simulink model "SystemModel"  (R2026a)
settings: Solver=FixedStepDiscrete  StopTime=inf  FixedStep=ts_system  EnableMultiTasking=on
StartFcn:
  | Simulink.sdi.setRecordData(false);
undefined symbols (not defined in the file): Battery, BCE12, BCE_Set_init, BMS_Controller_State, Cell10_P, Cell11_P, Cell12_P, Cell1_N, Cell1_P, Cell2_P, Cell3_P, Cell4_P, Cell5_P, Cell6_P, Cell7_P, Cell8_P, Cell9_P, Cell_Temperatures, Cell_Voltages, Charging_State, currentFactor, CV_Gain, Device_01, DiscIntNeverNeededParam, I_cc, MaxCellVoltThrsld, noCurrent, Ns_Module, NumModules, OverCellVoltageLimit, sg_bce, SOCInit, SRE, ts_controller, ts_system, UnderCellVoltageLimit, voltThreshold
libraries: slrealtimeethercatlib x99, fl_lib x65, nesl_utility x43, simulink x23, slrealtimeutilitieslib x13, sl_discontinuities x13, dspstat3 x12, canmsglib x11, speedgoatlib_IO611 x9, batt_lib x3, sharedTrackingLibrary x2, BatteryModuleLibrary_12Cells_lib x1
(part 6 of 6)

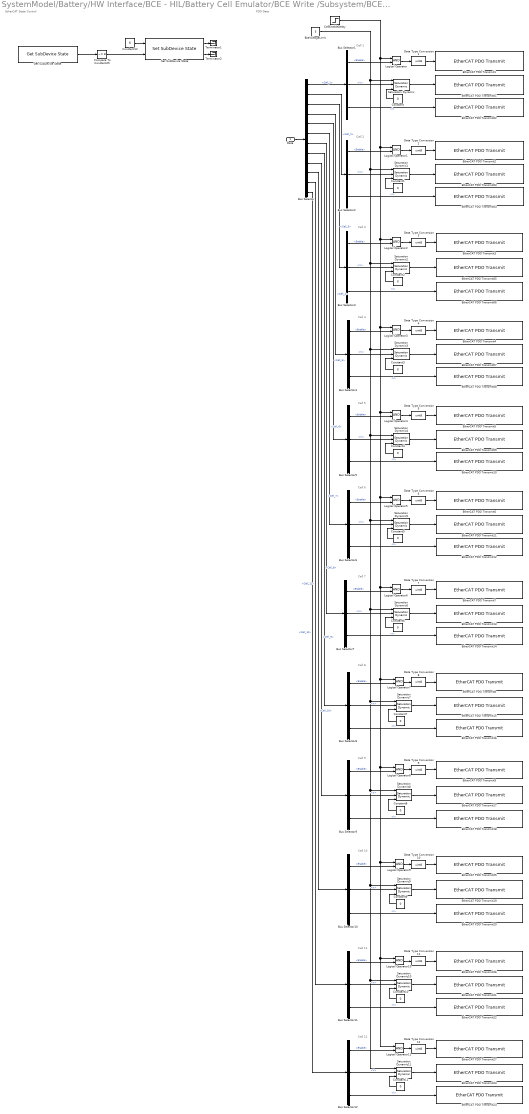
== system SystemModel/Battery/HW Interface/BCE - HIL/Battery Cell Emulator/BCE Write /Subsystem/BCE Write  ==
  note: EtherCAT State Control
  note: Cell 4
  note: Cell 8
  note: Cell 9
  note: Cell 1
  note: Cell 7
  note: PDO Data
  note: Cell 5
  note: Cell 3
  note: Cell 10
  note: Cell 6
  note: Cell 11
  note: Cell 12
  note: Cell 2
  Data : Inport  OutDataTypeStr=Bus: BCE_Set
  BceVoltageLimit : Constant  Value=5  SampleTime=0.001
  Bus Selector : BusSelector  OutputSignals=Cell_1,Cell_2,Cell_3,Cell_4,Cell_5,Cell_6,Cell_7,Cell_8,Cell_9,Cell_10,Cell_11,Cell_12
  Bus Selector{1..12} (12 alike) : BusSelector  OutputSignals=Enable,V,I
  CellEnableDelay : Step  Time=2  SampleTime=0.001
  Compare To Constant25 : simulink/Logic and Bit Operations/Compare To Constant  relop=~=  const=8  OutDataTypeStr=boolean
  Constant{,1..11} (12 alike) : Constant  Value=0
  Constant12 : Constant  Value=8  OutDataTypeStr=int32
  Data Type Conversion{1..12} (12 alike) : DataTypeConversion  OutDataTypeStr=uint8  SaturateOnIntegerOverflow=off  RndMeth=Floor
  EtherCAT PDO Transmit01 : slrealtimeethercatlib/EtherCAT PDO Transmit  Priority=3  sig_name=Device_01 (BCE12-0505).Rx_Cell_01.setVoltage  sig_offset=8  sig_type=single  type_size=32  sig_dim=1  device_id=0  sample_time=0.001000
  EtherCAT PDO Transmit02 : slrealtimeethercatlib/EtherCAT PDO Transmit  Priority=3  sig_name=Device_01 (BCE12-0505).Rx_Cell_01.setCurrent  sig_offset=40  sig_type=single  type_size=32  sig_dim=1  device_id=0  sample_time=0.001000
  EtherCAT PDO Transmit03 : slrealtimeethercatlib/EtherCAT PDO Transmit  Priority=3  sig_name=Device_01 (BCE12-0505).Rx_Cell_02.setVoltage  sig_offset=80  sig_type=single  type_size=32  sig_dim=1  device_id=0  sample_time=0.001000
  EtherCAT PDO Transmit04 : slrealtimeethercatlib/EtherCAT PDO Transmit  Priority=3  sig_name=Device_01 (BCE12-0505).Rx_Cell_02.setCurrent  sig_offset=112  sig_type=single  type_size=32  sig_dim=1  device_id=0  sample_time=0.001000
  EtherCAT PDO Transmit05 : slrealtimeethercatlib/EtherCAT PDO Transmit  Priority=3  sig_name=Device_01 (BCE12-0505).Rx_Cell_03.setVoltage  sig_offset=152  sig_type=single  type_size=32  sig_dim=1  device_id=0  sample_time=0.001000
  EtherCAT PDO Transmit06 : slrealtimeethercatlib/EtherCAT PDO Transmit  Priority=3  sig_name=Device_01 (BCE12-0505).Rx_Cell_03.setCurrent  sig_offset=184  sig_type=single  type_size=32  sig_dim=1  device_id=0  sample_time=0.001000
  EtherCAT PDO Transmit07 : slrealtimeethercatlib/EtherCAT PDO Transmit  Priority=3  sig_name=Device_01 (BCE12-0505).Rx_Cell_04.setVoltage  sig_offset=224  sig_type=single  type_size=32  sig_dim=1  device_id=0  sample_time=0.001000
  EtherCAT PDO Transmit08 : slrealtimeethercatlib/EtherCAT PDO Transmit  Priority=3  sig_name=Device_01 (BCE12-0505).Rx_Cell_04.setCurrent  sig_offset=256  sig_type=single  type_size=32  sig_dim=1  device_id=0  sample_time=0.001000
  EtherCAT PDO Transmit09 : slrealtimeethercatlib/EtherCAT PDO Transmit  Priority=3  sig_name=Device_01 (BCE12-0505).Rx_Cell_05.setVoltage  sig_offset=296  sig_type=single  type_size=32  sig_dim=1  device_id=0  sample_time=0.001000
  EtherCAT PDO Transmit1 : slrealtimeethercatlib/EtherCAT PDO Transmit  Priority=3  sig_name=Device_01 (BCE12-0505).Rx_Cell_01.enableCell  sig_offset=0  sig_type=uint8  type_size=8  sig_dim=1  device_id=0  sample_time=0.001000
  EtherCAT PDO Transmit10 : slrealtimeethercatlib/EtherCAT PDO Transmit  Priority=3  sig_name=Device_01 (BCE12-0505).Rx_Cell_05.setCurrent  sig_offset=328  sig_type=single  type_size=32  sig_dim=1  device_id=0  sample_time=0.001000
  EtherCAT PDO Transmit11 : slrealtimeethercatlib/EtherCAT PDO Transmit  Priority=3  sig_name=Device_01 (BCE12-0505).Rx_Cell_06.setVoltage  sig_offset=368  sig_type=single  type_size=32  sig_dim=1  device_id=0  sample_time=0.001000
  EtherCAT PDO Transmit12 : slrealtimeethercatlib/EtherCAT PDO Transmit  Priority=3  sig_name=Device_01 (BCE12-0505).Rx_Cell_06.setCurrent  sig_offset=400  sig_type=single  type_size=32  sig_dim=1  device_id=0  sample_time=0.001000
  EtherCAT PDO Transmit13 : slrealtimeethercatlib/EtherCAT PDO Transmit  Priority=3  sig_name=Device_01 (BCE12-0505).Rx_Cell_07.setVoltage  sig_offset=440  sig_type=single  type_size=32  sig_dim=1  device_id=0  sample_time=0.001000
  EtherCAT PDO Transmit14 : slrealtimeethercatlib/EtherCAT PDO Transmit  Priority=3  sig_name=Device_01 (BCE12-0505).Rx_Cell_07.setCurrent  sig_offset=472  sig_type=single  type_size=32  sig_dim=1  device_id=0  sample_time=0.001000
  EtherCAT PDO Transmit15 : slrealtimeethercatlib/EtherCAT PDO Transmit  Priority=3  sig_name=Device_01 (BCE12-0505).Rx_Cell_08.setVoltage  sig_offset=512  sig_type=single  type_size=32  sig_dim=1  device_id=0  sample_time=0.001000
  EtherCAT PDO Transmit16 : slrealtimeethercatlib/EtherCAT PDO Transmit  Priority=3  sig_name=Device_01 (BCE12-0505).Rx_Cell_08.setCurrent  sig_offset=544  sig_type=single  type_size=32  sig_dim=1  device_id=0  sample_time=0.001000
  EtherCAT PDO Transmit17 : slrealtimeethercatlib/EtherCAT PDO Transmit  Priority=3  sig_name=Device_01 (BCE12-0505).Rx_Cell_09.setVoltage  sig_offset=584  sig_type=single  type_size=32  sig_dim=1  device_id=0  sample_time=0.001000
  EtherCAT PDO Transmit18 : slrealtimeethercatlib/EtherCAT PDO Transmit  Priority=3  sig_name=Device_01 (BCE12-0505).Rx_Cell_09.setCurrent  sig_offset=616  sig_type=single  type_size=32  sig_dim=1  device_id=0  sample_time=0.001000
  EtherCAT PDO Transmit19 : slrealtimeethercatlib/EtherCAT PDO Transmit  Priority=3  sig_name=Device_01 (BCE12-0505).Rx_Cell_10.setVoltage  sig_offset=656  sig_type=single  type_size=32  sig_dim=1  device_id=0  sample_time=0.001000
  EtherCAT PDO Transmit2 : slrealtimeethercatlib/EtherCAT PDO Transmit  Priority=3  sig_name=Device_01 (BCE12-0505).Rx_Cell_02.enableCell  sig_offset=72  sig_type=uint8  type_size=8  sig_dim=1  device_id=0  sample_time=0.001000
  EtherCAT PDO Transmit20 : slrealtimeethercatlib/EtherCAT PDO Transmit  Priority=3  sig_name=Device_01 (BCE12-0505).Rx_Cell_10.setCurrent  sig_offset=688  sig_type=single  type_size=32  sig_dim=1  device_id=0  sample_time=0.001000
  EtherCAT PDO Transmit21 : slrealtimeethercatlib/EtherCAT PDO Transmit  Priority=3  sig_name=Device_01 (BCE12-0505).Rx_Cell_11.setVoltage  sig_offset=728  sig_type=single  type_size=32  sig_dim=1  device_id=0  sample_time=0.001000
  EtherCAT PDO Transmit22 : slrealtimeethercatlib/EtherCAT PDO Transmit  Priority=3  sig_name=Device_01 (BCE12-0505).Rx_Cell_11.setCurrent  sig_offset=760  sig_type=single  type_size=32  sig_dim=1  device_id=0  sample_time=0.001000
  EtherCAT PDO Transmit23 : slrealtimeethercatlib/EtherCAT PDO Transmit  Priority=3  sig_name=Device_01 (BCE12-0505).Rx_Cell_12.setVoltage  sig_offset=800  sig_type=single  type_size=32  sig_dim=1  device_id=0  sample_time=0.001000
  EtherCAT PDO Transmit24 : slrealtimeethercatlib/EtherCAT PDO Transmit  Priority=3  sig_name=Device_01 (BCE12-0505).Rx_Cell_12.setCurrent  sig_offset=832  sig_type=single  type_size=32  sig_dim=1  device_id=0  sample_time=0.001000
  EtherCAT PDO Transmit25 : slrealtimeethercatlib/EtherCAT PDO Transmit  Priority=3  sig_name=Device_01 (BCE12-0505).Rx_Cell_10.enableCell  sig_offset=648  sig_type=uint8  type_size=8  sig_dim=1  device_id=0  sample_time=0.001000
  EtherCAT PDO Transmit26 : slrealtimeethercatlib/EtherCAT PDO Transmit  Priority=3  sig_name=Device_01 (BCE12-0505).Rx_Cell_11.enableCell  sig_offset=720  sig_type=uint8  type_size=8  sig_dim=1  device_id=0  sample_time=0.001000
  EtherCAT PDO Transmit27 : slrealtimeethercatlib/EtherCAT PDO Transmit  Priority=3  sig_name=Device_01 (BCE12-0505).Rx_Cell_12.enableCell  sig_offset=792  sig_type=uint8  type_size=8  sig_dim=1  device_id=0  sample_time=0.001000
  EtherCAT PDO Transmit3 : slrealtimeethercatlib/EtherCAT PDO Transmit  Priority=3  sig_name=Device_01 (BCE12-0505).Rx_Cell_03.enableCell  sig_offset=144  sig_type=uint8  type_size=8  sig_dim=1  device_id=0  sample_time=0.001000
  EtherCAT PDO Transmit4 : slrealtimeethercatlib/EtherCAT PDO Transmit  Priority=3  sig_name=Device_01 (BCE12-0505).Rx_Cell_04.enableCell  sig_offset=216  sig_type=uint8  type_size=8  sig_dim=1  device_id=0  sample_time=0.001000
  EtherCAT PDO Transmit5 : slrealtimeethercatlib/EtherCAT PDO Transmit  Priority=3  sig_name=Device_01 (BCE12-0505).Rx_Cell_05.enableCell  sig_offset=288  sig_type=uint8  type_size=8  sig_dim=1  device_id=0  sample_time=0.001000
  EtherCAT PDO Transmit6 : slrealtimeethercatlib/EtherCAT PDO Transmit  Priority=3  sig_name=Device_01 (BCE12-0505).Rx_Cell_06.enableCell  sig_offset=360  sig_type=uint8  type_size=8  sig_dim=1  device_id=0  sample_time=0.001000
  EtherCAT PDO Transmit7 : slrealtimeethercatlib/EtherCAT PDO Transmit  Priority=3  sig_name=Device_01 (BCE12-0505).Rx_Cell_07.enableCell  sig_offset=432  sig_type=uint8  type_size=8  sig_dim=1  device_id=0  sample_time=0.001000
  EtherCAT PDO Transmit8 : slrealtimeethercatlib/EtherCAT PDO Transmit  Priority=3  sig_name=Device_01 (BCE12-0505).Rx_Cell_08.enableCell  sig_offset=504  sig_type=uint8  type_size=8  sig_dim=1  device_id=0  sample_time=0.001000
  EtherCAT PDO Transmit9 : slrealtimeethercatlib/EtherCAT PDO Transmit  Priority=3  sig_name=Device_01 (BCE12-0505).Rx_Cell_09.enableCell  sig_offset=576  sig_type=uint8  type_size=8  sig_dim=1  device_id=0  sample_time=0.001000
  Get SubDevice State : slrealtimeethercatlib/Get SubDevice State  device_id=0  subdevice_name=Device_01 (BCE12-0505)  sample_time=0.001  subdevice_addr=1001  selected_subdevice=Term 1 (EK1100)  timeout=500  subdevice_found=1
  Logical Operator{,1..11} (12 alike) : Logic  AllPortsSameDT=off  OutDataTypeStr=boolean
  Saturation Dynamic{,1..11} (12 alike) : sl_discontinuities/Saturation Dynamic  OutMin=[]  OutMax=[]  OutDataTypeStr=Inherit: Same as second input  OutDataType=fixdt(1, 16)  OutScaling=2^-10  DoSatur=off
  Set SubDevice State : slrealtimeethercatlib/Set SubDevice State  device_id=0  subdevice_name=Device_01 (BCE12-0505)  sample_time=0.001  subdevice_addr=1001  selected_subdevice=Term 1 (EK1100)  subdevice_found=1
  Terminator1 : Terminator
  Terminator2 : Terminator
  wires:
  Logical Operator11/1 -> Data Type Conversion12/1
  Bus Selector12/1 -> Logical Operator11/2  "<Enable>"
  Logical Operator10/1 -> Data Type Conversion11/1
  Bus Selector11/1 -> Logical Operator10/2  "<Enable>"
  Logical Operator9/1 -> Data Type Conversion10/1
  Bus Selector10/1 -> Logical Operator9/2  "<Enable>"
  Logical Operator8/1 -> Data Type Conversion9/1
  Bus Selector9/1 -> Logical Operator8/2  "<Enable>"
  Logical Operator7/1 -> Data Type Conversion8/1
  Bus Selector8/1 -> Logical Operator7/2  "<Enable>"
  Logical Operator6/1 -> Data Type Conversion7/1
  Bus Selector7/1 -> Logical Operator6/2  "<Enable>"
  Logical Operator5/1 -> Data Type Conversion6/1
  Bus Selector6/1 -> Logical Operator5/2  "<Enable>"
  Logical Operator4/1 -> Data Type Conversion5/1
  Bus Selector5/1 -> Logical Operator4/2  "<Enable>"
  Logical Operator3/1 -> Data Type Conversion4/1
  Bus Selector4/1 -> Logical Operator3/2  "<Enable>"
  Logical Operator2/1 -> Data Type Conversion3/1
  Bus Selector3/1 -> Logical Operator2/2  "<Enable>"
  Logical Operator1/1 -> Data Type Conversion2/1
  Bus Selector2/1 -> Logical Operator1/2  "<Enable>"
  Logical Operator/1 -> Data Type Conversion1/1
  Bus Selector1/1 -> Logical Operator/2  "<Enable>"
  CellEnableDelay/1 -> Logical Operator/1, Logical Operator1/1, Logical Operator2/1, Logical Operator3/1, Logical Operator4/1, Logical Operator5/1, Logical Operator6/1, Logical Operator7/1, Logical Operator8/1, Logical Operator9/1, Logical Operator10/1, Logical Operator11/1
  Constant12/1 -> Set SubDevice State/1
  Compare To Constant25/1 -> Set SubDevice State/2
  Set SubDevice State/1 -> Terminator1/1
  Set SubDevice State/2 -> Terminator2/1
  Get SubDevice State/1 -> Compare To Constant25/1
  Saturation Dynamic11/1 -> EtherCAT PDO Transmit23/1
  Constant11/1 -> Saturation Dynamic11/3
  Saturation Dynamic10/1 -> EtherCAT PDO Transmit21/1
  Constant10/1 -> Saturation Dynamic10/3
  Saturation Dynamic9/1 -> EtherCAT PDO Transmit19/1
  Constant9/1 -> Saturation Dynamic9/3
  Saturation Dynamic8/1 -> EtherCAT PDO Transmit17/1
  Constant8/1 -> Saturation Dynamic8/3
  Saturation Dynamic7/1 -> EtherCAT PDO Transmit15/1
  Constant7/1 -> Saturation Dynamic7/3
  Saturation Dynamic6/1 -> EtherCAT PDO Transmit13/1
  Constant6/1 -> Saturation Dynamic6/3
  Saturation Dynamic5/1 -> EtherCAT PDO Transmit11/1
  Constant5/1 -> Saturation Dynamic5/3
  Saturation Dynamic4/1 -> EtherCAT PDO Transmit09/1
  Constant4/1 -> Saturation Dynamic4/3
  Saturation Dynamic3/1 -> EtherCAT PDO Transmit07/1
  Constant3/1 -> Saturation Dynamic3/3
  Saturation Dynamic2/1 -> EtherCAT PDO Transmit05/1
  Constant2/1 -> Saturation Dynamic2/3
  Saturation Dynamic1/1 -> EtherCAT PDO Transmit03/1
  Constant1/1 -> Saturation Dynamic1/3
  BceVoltageLimit/1 -> Saturation Dynamic1/1, Saturation Dynamic2/1, Saturation Dynamic3/1, Saturation Dynamic4/1, Saturation Dynamic5/1, Saturation Dynamic6/1, Saturation Dynamic7/1, Saturation Dynamic8/1, Saturation Dynamic9/1, Saturation Dynamic10/1, Saturation Dynamic11/1, Saturation Dynamic/1
  Constant/1 -> Saturation Dynamic/3
  Saturation Dynamic/1 -> EtherCAT PDO Transmit01/1
  Bus Selector6/3 -> EtherCAT PDO Transmit12/1  "<I>"
  Bus Selector/4 -> Bus Selector4/1  "<Cell_4>"
  Data Type Conversion7/1 -> EtherCAT PDO Transmit7/1
  Bus Selector11/3 -> EtherCAT PDO Transmit22/1  "<I>"
  Bus Selector9/3 -> EtherCAT PDO Transmit18/1  "<I>"
  Bus Selector/8 -> Bus Selector8/1  "<Cell_8>"
  Bus Selector8/2 -> Saturation Dynamic7/2  "<V>"
  Bus Selector5/2 -> Saturation Dynamic4/2  "<V>"
  Data Type Conversion11/1 -> EtherCAT PDO Transmit26/1
  Bus Selector5/3 -> EtherCAT PDO Transmit10/1  "<I>"
  Data/1 -> Bus Selector/1
  Bus Selector10/3 -> EtherCAT PDO Transmit20/1  "<I>"
  Bus Selector/11 -> Bus Selector11/1  "<Cell_11>"
  Bus Selector3/2 -> Saturation Dynamic2/2  "<V>"
  Bus Selector2/3 -> EtherCAT PDO Transmit04/1  "<I>"
  Bus Selector10/2 -> Saturation Dynamic9/2  "<V>"
  Bus Selector12/3 -> EtherCAT PDO Transmit24/1  "<I>"
  Bus Selector/5 -> Bus Selector5/1  "<Cell_5>"
  Bus Selector/10 -> Bus Selector10/1  "<Cell_10>"
  Bus Selector1/3 -> EtherCAT PDO Transmit02/1  "<I>"
  Data Type Conversion3/1 -> EtherCAT PDO Transmit3/1
  Bus Selector4/2 -> Saturation Dynamic3/2  "<V>"
  Bus Selector6/2 -> Saturation Dynamic5/2  "<V>"
  Bus Selector3/3 -> EtherCAT PDO Transmit06/1  "<I>"
  Bus Selector/12 -> Bus Selector12/1  "<Cell_12>"
  Bus Selector4/3 -> EtherCAT PDO Transmit08/1  "<I>"
  Data Type Conversion1/1 -> EtherCAT PDO Transmit1/1
  Data Type Conversion10/1 -> EtherCAT PDO Transmit25/1
  Data Type Conversion12/1 -> EtherCAT PDO Transmit27/1
  Data Type Conversion5/1 -> EtherCAT PDO Transmit5/1
  Data Type Conversion9/1 -> EtherCAT PDO Transmit9/1
  Data Type Conversion6/1 -> EtherCAT PDO Transmit6/1
  Data Type Conversion4/1 -> EtherCAT PDO Transmit4/1
  Bus Selector/9 -> Bus Selector9/1  "<Cell_9>"
  Bus Selector7/3 -> EtherCAT PDO Transmit14/1  "<I>"
  Bus Selector7/2 -> Saturation Dynamic6/2  "<V>"
  Data Type Conversion2/1 -> EtherCAT PDO Transmit2/1
  Bus Selector/6 -> Bus Selector6/1  "<Cell_6>"
  Bus Selector/2 -> Bus Selector2/1  "<Cell_2>"
  Bus Selector1/2 -> Saturation Dynamic/2  "<V>"
  Bus Selector/3 -> Bus Selector3/1  "<Cell_3>"
  Bus Selector8/3 -> EtherCAT PDO Transmit16/1  "<I>"
  Bus Selector/1 -> Bus Selector1/1  "<Cell_1>"
  Bus Selector11/2 -> Saturation Dynamic10/2  "<V>"
  Bus Selector/7 -> Bus Selector7/1  "<Cell_7>"
  Bus Selector2/2 -> Saturation Dynamic1/2  "<V>"
  Bus Selector12/2 -> Saturation Dynamic11/2  "<V>"
  Bus Selector9/2 -> Saturation Dynamic8/2  "<V>"
  Data Type Conversion8/1 -> EtherCAT PDO Transmit8/1

== stateflow chart SystemModel/BMS/MIL/Controller/BMS State Machine/State_Machine ==
  settings: updateMethod=DISCRETE  sampleTime=ts_controller
  state MainStateMachine [parallel]
    settings: executionOrder=1
    state Standby
      en:
      BMS_State = ...
      BMS_Controller_State.BMS_Idle;
    state Charging
      en:
      BMS_State = BMS_Controller_State.BMS_Charging;
      state Init_Mode
        en:
        ChargeModeReq = Charging_State.Init;
        ChargeCurrentReq = noCurrent;
      state CC_Mode
        en:
        ChargeModeReq = Charging_State.CC;
        du:
        ChargeCurrentReq = min(I_cc,ChargeCurrentLimit);
      state CV_Mode
        en:
        ChargeModeReq = Charging_State.CV;
        du:
        ChargeCurrentReq = ChargeCurrentReq - CV_Gain*(MaxCellVolt - MaxCellVoltThrsld);
        ChargeCurrentReq = min(ChargeCurrentReq, ChargeCurrentLimit);
      (default) -> Init_Mode
      CV_Mode -> Init_Mode : [State_Request ~= SRE.Charging || ...
          | ChargeCurrentReq <= (I_cc/currentFactor)]
      CC_Mode -> Init_Mode [order 1] : [State_Request ~= ...
          | SRE.Charging]
      Init_Mode -> CC_Mode : [State_Request == SRE.Charging && ...
          | MaxCellVolt < voltThreshold]
      CC_Mode -> CV_Mode [order 2] : [MaxCellVolt>=...
          | MaxCellVoltThrsld]
    state Driving
      en:
      BMS_State = ...
      BMS_Controller_State.BMS_Driving;
    state Fault
      en,du:
      BMS_State = ...
      BMS_Controller_State.BMS_Fault;
    (default) -> Standby
    Standby -> Fault [order 1] : [FaultPresent == true]
    Standby -> Charging [order 2] : [State_Request == SRE.Charging]
    (junction 699) -> Standby : [after(3,sec)]
    Charging -> Standby [order 3] : [State_Request ~= SRE.Charging]
    Standby -> Driving [order 3] : [State_Request == SRE.Driving]
    Driving -> Standby [order 3] : [State_Request ~= SRE.Driving]
    Driving -> Charging [order 2] : [State_Request == SRE.Charging]
    Charging -> Driving [order 2] : [State_Request == SRE.Driving]
    Fault -> (junction 699) : [[FaultPresent == false && Fault_Reset_Enable]]
    Driving -> Fault [order 1] : [FaultPresent]
    Charging -> Fault [order 1] : [FaultPresent]{ChargeCurrentReq = single(0);}
  state FaultMonitoring [parallel]
    settings: executionOrder=2
    state MonitorCellVoltage [parallel]
      settings: executionOrder=1
      state OverVoltageFault
        en:
        FaultPresent = true;
        Fault_out.OverVolt = true;
        du:
        MaxCellVolt = max(Cell_Voltages);
      state NoCellVoltFault
        en,du:
        MaxCellVolt = max(Cell_Voltages);
        MinCellVolt = min(Cell_Voltages);
      state UnderVoltageFault
        en:
        FaultPresent = true;
        Fault_out.UnderVolt = true;
        du:
        MinCellVolt = min(Cell_Voltages);
      OverVoltageFault -> (junction 687) : [MaxCellVolt < OverCellVoltageLimit && ...
          | Fault_Reset_Enable ...
          | ]{Fault_out.OverVolt=false; ...
          | FaultPresent = false;}
      (junction 695) -> OverVoltageFault : [after(100,msec)]
      NoCellVoltFault -> (junction 695) [order 1] : [MaxCellVolt >= ...
          | OverCellVoltageLimit]
      (junction 687) -> NoCellVoltFault : [after(3,sec)]
      (default) -> NoCellVoltFault : {FaultPresent = false;
          | Fault_out.OverVolt = false;
          | Fault_out.UnderVolt = false;}
      NoCellVoltFault -> (junction 697) [order 2] : [MinCellVolt <=...
          |  UnderCellVoltageLimit]
      (junction 685) -> NoCellVoltFault : [after(3,sec)]
      (junction 697) -> UnderVoltageFault : [after(100,msec)]
      UnderVoltageFault -> (junction 685) : [MinCellVolt > UnderCellVoltageLimit && ...
          | Fault_Reset_Enable] ...
          | {Fault_out.UnderVolt=false; ...
          | FaultPresent = false;}
    state MonitorCurrLim [parallel]
      settings: executionOrder=3
      state NoCurrLimFault
        en:
        FaultPresent = false;
        Fault_out.OverCurrent = false;
      state OverCurrentFault
        en:
        FaultPresent = true;
        Fault_out.OverCurrent=true;
      (default) -> NoCurrLimFault : {FaultPresent = false;
          | Fault_out.OverCurrent=false;}
      (junction 678) -> NoCurrLimFault : [after(3,sec)]
      NoCurrLimFault -> (junction 675) : [((DischargeCurrentLimit - Pack_Current) > single(0.2) && ...
          | BMS_State == BMS_Controller_State.BMS_Driving) || ...
          | ((Pack_Current - ChargeCurrentLimit) > single(0.2) && ...
          | BMS_State == BMS_Controller_State.BMS_Charging)]
      OverCurrentFault -> (junction 678) : [(Pack_Current >= DischargeCurrentLimit || ...
          |  Pack_Current <= ChargeCurrentLimit) && ...
          | Fault_Reset_Enable]
      (junction 675) -> OverCurrentFault : [after(100,msec)]
    state MonitorCellTemp [parallel]
      settings: executionOrder=2
      state HighTemperatureFault
        en:
        FaultPresent = true;
        Fault_out.HighTemp = true;
        du:
        MaxCellTemp = max(Cell_Temperatures);
      state NoCellTempFault
        en,du:
        MaxCellTemp = max(Cell_Temperatures);
        MinCellTemp = min(Cell_Temperatures);
      state LowTemperatureFault
        en:
        FaultPresent = true;
        Fault_out.LowTemp = true;
        du:
        MinCellTemp = min(Cell_Temperatures);
      HighTemperatureFault -> (junction 680) : [MaxCellTemp < HighTempLimit && ...
          | Fault_Reset_Enable] ...
          | {Fault_out.HighTemp=false; FaultPresent = false;}
      (junction 689) -> HighTemperatureFault : [after(100,msec)]
      (junction 680) -> NoCellTempFault : [after(3,sec)]
      NoCellTempFault -> (junction 689) [order 1] : [MaxCellTemp >= HighTempLimit]
      (default) -> NoCellTempFault : {FaultPresent = false;
          | Fault_out.HighTemp = false;
          | Fault_out.LowTemp = false;}
      (junction 682) -> NoCellTempFault : [after(3,sec)]
      NoCellTempFault -> (junction 691) [order 2] : [MinCellTemp <= LowTempLimit]
      LowTemperatureFault -> (junction 682) : [MinCellTemp > LowTempLimit && ...
          | Fault_Reset_Enable ] ...
          | {Fault_out.LowTemp=false; FaultPresent = false;}
      (junction 691) -> LowTemperatureFault : [after(100,msec)]
  data: DischargeCurrentLimit input single; ChargeCurrentLimit input single; State_Request input; Cell_Voltages input single; Pack_Voltage input single; Cell_Temperatures input single; Pack_Current input single; ChargeCurrentReq output; I_cc parameter; MaxCellVoltThrsld parameter; FaultPresent local; MaxCellTemp local; OverCellVoltageLimit parameter; UnderCellVoltageLimit parameter; MinCellTemp local; CV_Gain parameter; MonitorCurrLimMode local Enum: MonitorCurrLimModeType; MonitorCellVoltageMode local Enum: MonitorCellVoltageModeType; MonitorCellTempMode local Enum: MonitorCellTempModeType; Fault_out output Bus: Faults; voltThreshold parameter single; currentFactor parameter single; noCurrent parameter single; Fault_Reset_Enable input boolean; ChargeModeReq output Enum: Charging_State =Charging_State.Init; BMS_State output Enum: BMS_Controller_State =BMS_Controller_State.BMS_Idle; MaxCellVolt local; MinCellVolt local; HighTempLimit local =single(323.15); LowTempLimit local =single(278.15)

== stateflow chart SystemModel/BMS/MIL/Controller/Balancing Logic/Balancing ==
  settings: updateMethod=DISCRETE
  state BalancingOFF
    en:
    Bal_Cmd(:,:) = false;
    en,du:
    MaxCellVolt = max(CellVoltages);
    MinCellVolt = min(CellVoltages);
    DeltaCellVolt = MaxCellVolt - MinCellVolt;
  state BalancingON
    en, du:
    MaxCellVolt = max(CellVoltages);
    MinCellVolt = min(CellVoltages);
    DeltaCellVolt = MaxCellVolt - MinCellVolt;
    state BalActive
      en, du:
      Bal_Cmd = ((CellVoltages - MinCellVolt) > TargetDeltaV)';
      flgBalCompl = all(~Bal_Cmd);
    state BalNotActive
    (default) -> BalActive
    BalNotActive -> BalActive [order 1] : [after(BalNotActWait,sec) && ...
        | DeltaCellVolt > TargetDeltaV]
    BalActive -> BalNotActive : [flgBalCompl]
  note: "Copyright 2018 - 2019 The MathWorks, Inc."
  (default) -> BalancingOFF : {flgBalCompl = true;}
  BalancingOFF -> BalancingON : [flgEnBalancing && ...
      | BMS_State ~= BMS_Controller_State.BMS_Driving && ...
      | BMS_State ~= BMS_Controller_State.BMS_Fault && ...
      | after(BalOffWait,sec) && ...
      | DeltaCellVolt > TargetDeltaV]
  BalancingON -> BalancingOFF : [BMS_State == BMS_Controller_State.BMS_Driving]
  BalNotActive -> BalancingOFF [order 2] : [after(BalOnWait,sec)]
  data: BMS_State input Enum: BMS_Controller_State; CellVoltages input single; Bal_Cmd output boolean size=[1,Ns_Module*NumModules] =boolean(zeros(1,Ns_Module*NumModules)); flgBalCompl local; BalNotActWait local =int16(10); BalOffWait local =int16(5); BalOnWait local =int16(20); flgEnBalancing local =boolean(1); DeltaCellVolt local single =single(0); MaxCellVolt local =single(4); MinCellVolt local =single(3); TargetDeltaV local =single(0.1)
